simulink model "temp_and_humd_sensor"  (R2017a)
settings: Solver=VariableStepAuto  StartTime=0.0  StopTime=20  RelTol=1e-3
settings Model: Creator=Mads  LastModifiedBy=Mads

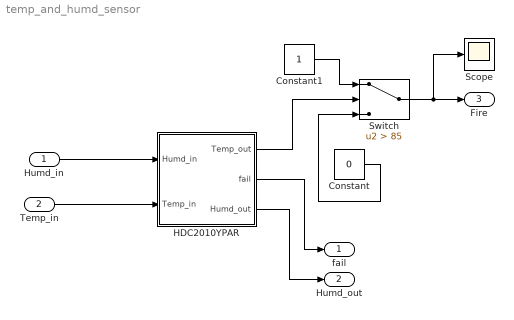
== system temp_and_humd_sensor ==
  Humd_in : Inport
  Temp_in : Inport  Port=2
  Constant : Constant  Value=0
  Constant1 : Constant
  HDC2010YPAR : Subsystem
  Scope : Scope
  Switch : Switch  Criteria=u2 > Threshold  Threshold=85
  fail : Outport
  Humd_out : Outport  Port=2
  Fire : Outport  Port=3
  wires:
  Humd_in/1 -> HDC2010YPAR/1(Humd_in)
  Temp_in/1 -> HDC2010YPAR/2(Temp_in)
  HDC2010YPAR/2(fail) -> fail/1
  HDC2010YPAR/3(Humd_out) -> Humd_out/1
  HDC2010YPAR/1(Temp_out) -> Switch/2
  Constant1/1 -> Switch/1
  Constant/1 -> Switch/3
  Switch/1 -> Scope/1, Fire/1

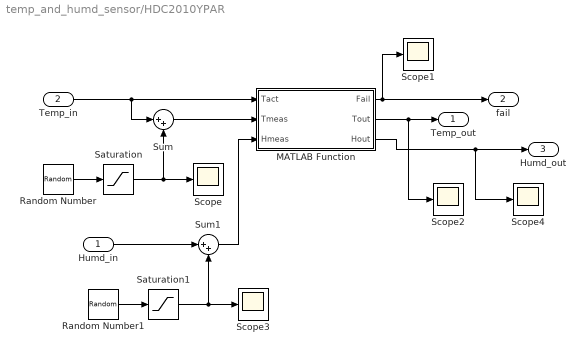
== system temp_and_humd_sensor/HDC2010YPAR ==
  Humd_in : Inport
  Temp_in : Inport  Port=2
  MATLAB Function : MATLAB Function  TreatAsAtomicUnit=on
  Random Number : RandomNumber  Variance=0.1  SampleTime=1
  Random Number1 : RandomNumber  Variance=2  SampleTime=1
  Saturation : Saturate  UpperLimit=0.2  LowerLimit=-0.2
  Saturation1 : Saturate  UpperLimit=2  LowerLimit=-2
  Scope{,1..4} (5 alike) : Scope
  Sum : Sum  Inputs=|++
  Sum1 : Sum  Inputs=|++
  Temp_out : Outport
  fail : Outport  Port=2
  Humd_out : Outport  Port=3
  wires:
  MATLAB Function/2(Tout) -> Scope2/1, Temp_out/1
  MATLAB Function/3(Hout) -> Humd_out/1, Scope4/1
  Saturation/1 -> Scope/1, Sum/2
  Sum/1 -> MATLAB Function/2(Tmeas)
  Random Number/1 -> Saturation/1
  Random Number1/1 -> Saturation1/1
  Saturation1/1 -> Scope3/1, Sum1/2
  Temp_in/1 -> MATLAB Function/1(Tact), Sum/1
  MATLAB Function/1(Fail) -> fail/1, Scope1/1
  Sum1/1 -> MATLAB Function/3(Hmeas)
  Humd_in/1 -> Sum1/1

== matlab function temp_and_humd_sensor/HDC2010YPAR/MATLAB Function ==
  data: Tact input; Fail output; Tmeas input; Tout output; Hmeas input; Hout output
function [Fail,Tout,Hout]= sensorFail(Tact,Tmeas,Hmeas)
    if ( Tact < -40 ) || (Tact > 125 ) 
        Fail = -1 ; % outside operating temp, sensor failure 
        Tout = 0 ;
        Hout = 0 ;
    else 
        Fail = 0 ; % within operating temp 
        Tout = Tmeas ;
        Hout = Hmeas ;
    end
end
